simulink model "BloquesParkInversa"  (R2023b)
settings: Solver=VariableStepAuto  StartTime=0.0  StopTime=10.0  RelTol=1e-3
values from neighbouring files (symbols this model uses):
  P_p = 3    [Parametros.m]
settings Model: Creator=Home  LastModifiedBy=Home

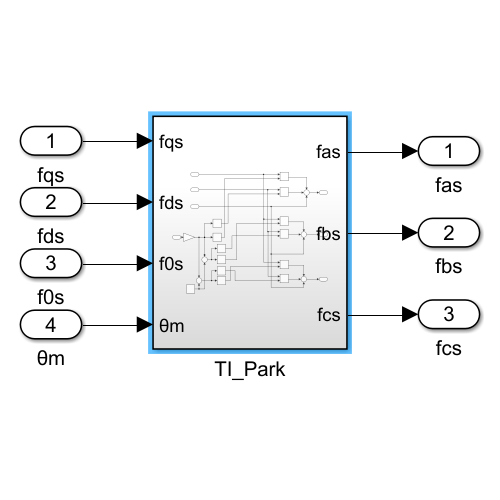
[thumbnail: Simulink's stored preview of the top-level diagram]
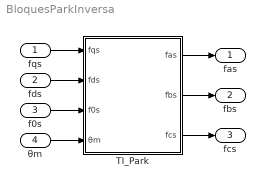
== system BloquesParkInversa ==
  fqs : Inport
  fds : Inport  Port=2
  f0s : Inport  Port=3
  θm : Inport  Port=4
  TI_Park : Subsystem
  fas : Outport
  fbs : Outport  Port=2
  fcs : Outport  Port=3
  wires:
  fqs/1 -> TI_Park/1(fqs)
  fds/1 -> TI_Park/2(fds)
  f0s/1 -> TI_Park/3(f0s)
  θm/1 -> TI_Park/4(θm)
  TI_Park/1(fas) -> fas/1
  TI_Park/2(fbs) -> fbs/1
  TI_Park/3(fcs) -> fcs/1

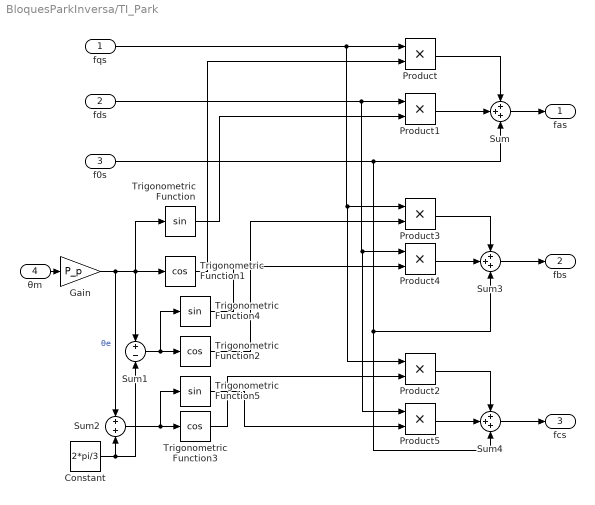
== system BloquesParkInversa/TI_Park ==
  fqs : Inport
  fds : Inport  Port=2
  f0s : Inport  Port=3
  θm : Inport  Port=4
  Constant : Constant  Value=2*pi/3
  Gain : Gain  Gain=P_p
  Product{,1..5} (6 alike) : Product
  Sum : Sum  Inputs=+++
  Sum1 : Sum  Inputs=+-
  Sum2 : Sum
  Sum3 : Sum  Inputs=+++
  Sum4 : Sum  Inputs=+++
  Trigonometric Function : Trigonometry
  Trigonometric Function1 : Trigonometry  Operator=cos
  Trigonometric Function2 : Trigonometry  Operator=cos
  Trigonometric Function3 : Trigonometry  Operator=cos
  Trigonometric Function4 : Trigonometry
  Trigonometric Function5 : Trigonometry
  fas : Outport
  fbs : Outport  Port=2
  fcs : Outport  Port=3
  wires:
  Constant/1 -> Sum2/2, Sum1/2
  Product1/1 -> Sum/2
  Trigonometric Function2/1 -> Product3/2
  θm/1 -> Gain/1
  Trigonometric Function5/1 -> Product5/2
  fds/1 -> Product1/1, Product5/1, Product4/1
  f0s/1 -> Sum/3, Sum3/3, Sum4/3
  Product3/1 -> Sum3/1
  fqs/1 -> Product/1, Product2/1, Product3/1
  Product2/1 -> Sum4/1
  Trigonometric Function1/1 -> Product/2
  Product/1 -> Sum/1
  Sum2/1 -> Trigonometric Function5/1, Trigonometric Function3/1
  Sum1/1 -> Trigonometric Function4/1, Trigonometric Function2/1
  Trigonometric Function/1 -> Product1/2
  Product4/1 -> Sum3/2
  Sum/1 -> fas/1
  Trigonometric Function3/1 -> Product2/2
  Product5/1 -> Sum4/2
  Trigonometric Function4/1 -> Product4/2
  Sum3/1 -> fbs/1
  Sum4/1 -> fcs/1
  Gain/1 -> Trigonometric Function/1, Sum1/1, Trigonometric Function1/1, Sum2/1  "θe"
